simulink subsystem "clarke"  (R2022b)
settings: Solver=VariableStepAuto  StartTime=0.0  StopTime=10.0  RelTol=1e-3
settings Model: Creator=jack  LastModifiedBy=jack

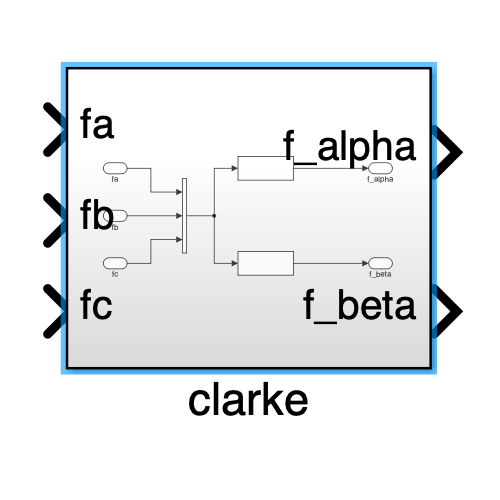
[thumbnail: Simulink's stored preview of the top-level diagram]
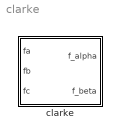
== system clarke ==
  clarke : Subsystem

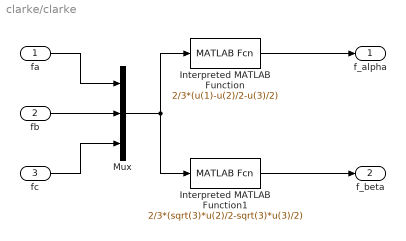
== system clarke/clarke ==
  fa : Inport
  fb : Inport  Port=2
  fc : Inport  Port=3
  Interpreted MATLAB Function : MATLABFcn  MATLABFcn=2/3*(u(1)-u(2)/2-u(3)/2)
  Interpreted MATLAB Function1 : MATLABFcn  MATLABFcn=2/3*(sqrt(3)*u(2)/2-sqrt(3)*u(3)/2)
  Mux : Mux  Inputs=3
  f_alpha : Outport
  f_beta : Outport  Port=2
  wires:
  Interpreted MATLAB Function/1 -> f_alpha/1
  fa/1 -> Mux/1
  Mux/1 -> Interpreted MATLAB Function1/1, Interpreted MATLAB Function/1
  Interpreted MATLAB Function1/1 -> f_beta/1
  fc/1 -> Mux/3
  fb/1 -> Mux/2
